simulink model "sdbe_10_11"  (R2012b)
settings: Solver=VariableStepDiscrete  SolverMode=SingleTasking  StartTime=0.0  StopTime=10000  RelTol=1e-3
PreLoadFcn:
  | counter_vals
undefined symbols (not defined in the file or in its folder): sfp
libraries: xbsIndex_r4 x8459, casper_library_misc x39, casper_library_delays x27, dspsigops x16, xps_library x10, r2dbe_vdif_lib x4, r2dbe_adc_lib x3, simulink x1
(part 61 of 72)

== system sdbe_10_11/get_data_from_pkt2/scope/quant11/is_positive ==
  d : Inport
  Reinterpret : xbsIndex_r4/Reinterpret  force_arith_type=on  arith_type=Unsigned  force_bin_pt=on  bin_pt=0  block_type=reinterpret
  not : xbsIndex_r4/Inverter  en=off  latency=0  dbl_ovrd=off  block_type=inv
  sgn : xbsIndex_r4/Slice  nbits=1  boolean_output=off  mode=Upper Bit Location + Width  bit1=0  base1=MSB of Input  bit0=0  base0=LSB of Input  dbl_ovrd=off  block_type=slice
  q : Outport
  wires:
  sgn/1 -> not/1
  Reinterpret/1 -> sgn/1
  d/1 -> Reinterpret/1
  not/1 -> q/1

== system sdbe_10_11/get_data_from_pkt2/scope/quant12/is_positive ==
  d : Inport
  Reinterpret : xbsIndex_r4/Reinterpret  force_arith_type=on  arith_type=Unsigned  force_bin_pt=on  bin_pt=0  block_type=reinterpret
  not : xbsIndex_r4/Inverter  en=off  latency=0  dbl_ovrd=off  block_type=inv
  sgn : xbsIndex_r4/Slice  nbits=1  boolean_output=off  mode=Upper Bit Location + Width  bit1=0  base1=MSB of Input  bit0=0  base0=LSB of Input  dbl_ovrd=off  block_type=slice
  q : Outport
  wires:
  not/1 -> q/1
  d/1 -> Reinterpret/1
  Reinterpret/1 -> sgn/1
  sgn/1 -> not/1

== system sdbe_10_11/get_data_from_pkt2/scope/quant13/is_positive ==
  d : Inport
  Reinterpret : xbsIndex_r4/Reinterpret  force_arith_type=on  arith_type=Unsigned  force_bin_pt=on  bin_pt=0  block_type=reinterpret
  not : xbsIndex_r4/Inverter  en=off  latency=0  dbl_ovrd=off  block_type=inv
  sgn : xbsIndex_r4/Slice  nbits=1  boolean_output=off  mode=Upper Bit Location + Width  bit1=0  base1=MSB of Input  bit0=0  base0=LSB of Input  dbl_ovrd=off  block_type=slice
  q : Outport
  wires:
  sgn/1 -> not/1
  Reinterpret/1 -> sgn/1
  d/1 -> Reinterpret/1
  not/1 -> q/1

== system sdbe_10_11/get_data_from_pkt2/scope/quant14/is_positive ==
  d : Inport
  Reinterpret : xbsIndex_r4/Reinterpret  force_arith_type=on  arith_type=Unsigned  force_bin_pt=on  bin_pt=0  block_type=reinterpret
  not : xbsIndex_r4/Inverter  en=off  latency=0  dbl_ovrd=off  block_type=inv
  sgn : xbsIndex_r4/Slice  nbits=1  boolean_output=off  mode=Upper Bit Location + Width  bit1=0  base1=MSB of Input  bit0=0  base0=LSB of Input  dbl_ovrd=off  block_type=slice
  q : Outport
  wires:
  sgn/1 -> not/1
  Reinterpret/1 -> sgn/1
  d/1 -> Reinterpret/1
  not/1 -> q/1

== system sdbe_10_11/get_data_from_pkt2/scope/quant15/is_positive ==
  d : Inport
  Reinterpret : xbsIndex_r4/Reinterpret  force_arith_type=on  arith_type=Unsigned  force_bin_pt=on  bin_pt=0  block_type=reinterpret
  not : xbsIndex_r4/Inverter  en=off  latency=0  dbl_ovrd=off  block_type=inv
  sgn : xbsIndex_r4/Slice  nbits=1  boolean_output=off  mode=Upper Bit Location + Width  bit1=0  base1=MSB of Input  bit0=0  base0=LSB of Input  dbl_ovrd=off  block_type=slice
  q : Outport
  wires:
  not/1 -> q/1
  d/1 -> Reinterpret/1
  Reinterpret/1 -> sgn/1
  sgn/1 -> not/1

== system sdbe_10_11/get_data_from_pkt2/scope/quant2/is_positive ==
  d : Inport
  Reinterpret : xbsIndex_r4/Reinterpret  force_arith_type=on  arith_type=Unsigned  force_bin_pt=on  bin_pt=0  block_type=reinterpret
  not : xbsIndex_r4/Inverter  en=off  latency=0  dbl_ovrd=off  block_type=inv
  sgn : xbsIndex_r4/Slice  nbits=1  boolean_output=off  mode=Upper Bit Location + Width  bit1=0  base1=MSB of Input  bit0=0  base0=LSB of Input  dbl_ovrd=off  block_type=slice
  q : Outport
  wires:
  sgn/1 -> not/1
  Reinterpret/1 -> sgn/1
  d/1 -> Reinterpret/1
  not/1 -> q/1

== system sdbe_10_11/get_data_from_pkt2/scope/quant3/is_positive ==
  d : Inport
  Reinterpret : xbsIndex_r4/Reinterpret  force_arith_type=on  arith_type=Unsigned  force_bin_pt=on  bin_pt=0  block_type=reinterpret
  not : xbsIndex_r4/Inverter  en=off  latency=0  dbl_ovrd=off  block_type=inv
  sgn : xbsIndex_r4/Slice  nbits=1  boolean_output=off  mode=Upper Bit Location + Width  bit1=0  base1=MSB of Input  bit0=0  base0=LSB of Input  dbl_ovrd=off  block_type=slice
  q : Outport
  wires:
  not/1 -> q/1
  d/1 -> Reinterpret/1
  Reinterpret/1 -> sgn/1
  sgn/1 -> not/1

== system sdbe_10_11/get_data_from_pkt2/scope/quant4/is_positive ==
  d : Inport
  Reinterpret : xbsIndex_r4/Reinterpret  force_arith_type=on  arith_type=Unsigned  force_bin_pt=on  bin_pt=0  block_type=reinterpret
  not : xbsIndex_r4/Inverter  en=off  latency=0  dbl_ovrd=off  block_type=inv
  sgn : xbsIndex_r4/Slice  nbits=1  boolean_output=off  mode=Upper Bit Location + Width  bit1=0  base1=MSB of Input  bit0=0  base0=LSB of Input  dbl_ovrd=off  block_type=slice
  q : Outport
  wires:
  sgn/1 -> not/1
  Reinterpret/1 -> sgn/1
  d/1 -> Reinterpret/1
  not/1 -> q/1

== system sdbe_10_11/get_data_from_pkt2/scope/quant5/is_positive ==
  d : Inport
  Reinterpret : xbsIndex_r4/Reinterpret  force_arith_type=on  arith_type=Unsigned  force_bin_pt=on  bin_pt=0  block_type=reinterpret
  not : xbsIndex_r4/Inverter  en=off  latency=0  dbl_ovrd=off  block_type=inv
  sgn : xbsIndex_r4/Slice  nbits=1  boolean_output=off  mode=Upper Bit Location + Width  bit1=0  base1=MSB of Input  bit0=0  base0=LSB of Input  dbl_ovrd=off  block_type=slice
  q : Outport
  wires:
  not/1 -> q/1
  d/1 -> Reinterpret/1
  Reinterpret/1 -> sgn/1
  sgn/1 -> not/1

== system sdbe_10_11/get_data_from_pkt2/scope/quant6/is_positive ==
  d : Inport
  Reinterpret : xbsIndex_r4/Reinterpret  force_arith_type=on  arith_type=Unsigned  force_bin_pt=on  bin_pt=0  block_type=reinterpret
  not : xbsIndex_r4/Inverter  en=off  latency=0  dbl_ovrd=off  block_type=inv
  sgn : xbsIndex_r4/Slice  nbits=1  boolean_output=off  mode=Upper Bit Location + Width  bit1=0  base1=MSB of Input  bit0=0  base0=LSB of Input  dbl_ovrd=off  block_type=slice
  q : Outport
  wires:
  not/1 -> q/1
  d/1 -> Reinterpret/1
  Reinterpret/1 -> sgn/1
  sgn/1 -> not/1

== system sdbe_10_11/get_data_from_pkt2/scope/quant7/is_positive ==
  d : Inport
  Reinterpret : xbsIndex_r4/Reinterpret  force_arith_type=on  arith_type=Unsigned  force_bin_pt=on  bin_pt=0  block_type=reinterpret
  not : xbsIndex_r4/Inverter  en=off  latency=0  dbl_ovrd=off  block_type=inv
  sgn : xbsIndex_r4/Slice  nbits=1  boolean_output=off  mode=Upper Bit Location + Width  bit1=0  base1=MSB of Input  bit0=0  base0=LSB of Input  dbl_ovrd=off  block_type=slice
  q : Outport
  wires:
  sgn/1 -> not/1
  Reinterpret/1 -> sgn/1
  d/1 -> Reinterpret/1
  not/1 -> q/1

== system sdbe_10_11/get_data_from_pkt2/scope/quant8/is_positive ==
  d : Inport
  Reinterpret : xbsIndex_r4/Reinterpret  force_arith_type=on  arith_type=Unsigned  force_bin_pt=on  bin_pt=0  block_type=reinterpret
  not : xbsIndex_r4/Inverter  en=off  latency=0  dbl_ovrd=off  block_type=inv
  sgn : xbsIndex_r4/Slice  nbits=1  boolean_output=off  mode=Upper Bit Location + Width  bit1=0  base1=MSB of Input  bit0=0  base0=LSB of Input  dbl_ovrd=off  block_type=slice
  q : Outport
  wires:
  sgn/1 -> not/1
  Reinterpret/1 -> sgn/1
  d/1 -> Reinterpret/1
  not/1 -> q/1

== system sdbe_10_11/get_data_from_pkt2/scope/quant9/is_positive ==
  d : Inport
  Reinterpret : xbsIndex_r4/Reinterpret  force_arith_type=on  arith_type=Unsigned  force_bin_pt=on  bin_pt=0  block_type=reinterpret
  not : xbsIndex_r4/Inverter  en=off  latency=0  dbl_ovrd=off  block_type=inv
  sgn : xbsIndex_r4/Slice  nbits=1  boolean_output=off  mode=Upper Bit Location + Width  bit1=0  base1=MSB of Input  bit0=0  base0=LSB of Input  dbl_ovrd=off  block_type=slice
  q : Outport
  wires:
  not/1 -> q/1
  d/1 -> Reinterpret/1
  Reinterpret/1 -> sgn/1
  sgn/1 -> not/1

== system sdbe_10_11/get_data_from_pkt3/scope/quant0/is_positive ==
  d : Inport
  Reinterpret : xbsIndex_r4/Reinterpret  force_arith_type=on  arith_type=Unsigned  force_bin_pt=on  bin_pt=0  block_type=reinterpret
  not : xbsIndex_r4/Inverter  en=off  latency=0  dbl_ovrd=off  block_type=inv
  sgn : xbsIndex_r4/Slice  nbits=1  boolean_output=off  mode=Upper Bit Location + Width  bit1=0  base1=MSB of Input  bit0=0  base0=LSB of Input  dbl_ovrd=off  block_type=slice
  q : Outport
  wires:
  sgn/1 -> not/1
  Reinterpret/1 -> sgn/1
  d/1 -> Reinterpret/1
  not/1 -> q/1

== system sdbe_10_11/get_data_from_pkt3/scope/quant1/is_positive ==
  d : Inport
  Reinterpret : xbsIndex_r4/Reinterpret  force_arith_type=on  arith_type=Unsigned  force_bin_pt=on  bin_pt=0  block_type=reinterpret
  not : xbsIndex_r4/Inverter  en=off  latency=0  dbl_ovrd=off  block_type=inv
  sgn : xbsIndex_r4/Slice  nbits=1  boolean_output=off  mode=Upper Bit Location + Width  bit1=0  base1=MSB of Input  bit0=0  base0=LSB of Input  dbl_ovrd=off  block_type=slice
  q : Outport
  wires:
  not/1 -> q/1
  d/1 -> Reinterpret/1
  Reinterpret/1 -> sgn/1
  sgn/1 -> not/1

== system sdbe_10_11/get_data_from_pkt3/scope/quant10/is_positive ==
  d : Inport
  Reinterpret : xbsIndex_r4/Reinterpret  force_arith_type=on  arith_type=Unsigned  force_bin_pt=on  bin_pt=0  block_type=reinterpret
  not : xbsIndex_r4/Inverter  en=off  latency=0  dbl_ovrd=off  block_type=inv
  sgn : xbsIndex_r4/Slice  nbits=1  boolean_output=off  mode=Upper Bit Location + Width  bit1=0  base1=MSB of Input  bit0=0  base0=LSB of Input  dbl_ovrd=off  block_type=slice
  q : Outport
  wires:
  sgn/1 -> not/1
  Reinterpret/1 -> sgn/1
  d/1 -> Reinterpret/1
  not/1 -> q/1

== system sdbe_10_11/get_data_from_pkt3/scope/quant11/is_positive ==
  d : Inport
  Reinterpret : xbsIndex_r4/Reinterpret  force_arith_type=on  arith_type=Unsigned  force_bin_pt=on  bin_pt=0  block_type=reinterpret
  not : xbsIndex_r4/Inverter  en=off  latency=0  dbl_ovrd=off  block_type=inv
  sgn : xbsIndex_r4/Slice  nbits=1  boolean_output=off  mode=Upper Bit Location + Width  bit1=0  base1=MSB of Input  bit0=0  base0=LSB of Input  dbl_ovrd=off  block_type=slice
  q : Outport
  wires:
  not/1 -> q/1
  d/1 -> Reinterpret/1
  Reinterpret/1 -> sgn/1
  sgn/1 -> not/1

== system sdbe_10_11/get_data_from_pkt3/scope/quant12/is_positive ==
  d : Inport
  Reinterpret : xbsIndex_r4/Reinterpret  force_arith_type=on  arith_type=Unsigned  force_bin_pt=on  bin_pt=0  block_type=reinterpret
  not : xbsIndex_r4/Inverter  en=off  latency=0  dbl_ovrd=off  block_type=inv
  sgn : xbsIndex_r4/Slice  nbits=1  boolean_output=off  mode=Upper Bit Location + Width  bit1=0  base1=MSB of Input  bit0=0  base0=LSB of Input  dbl_ovrd=off  block_type=slice
  q : Outport
  wires:
  sgn/1 -> not/1
  Reinterpret/1 -> sgn/1
  d/1 -> Reinterpret/1
  not/1 -> q/1

== system sdbe_10_11/get_data_from_pkt3/scope/quant13/is_positive ==
  d : Inport
  Reinterpret : xbsIndex_r4/Reinterpret  force_arith_type=on  arith_type=Unsigned  force_bin_pt=on  bin_pt=0  block_type=reinterpret
  not : xbsIndex_r4/Inverter  en=off  latency=0  dbl_ovrd=off  block_type=inv
  sgn : xbsIndex_r4/Slice  nbits=1  boolean_output=off  mode=Upper Bit Location + Width  bit1=0  base1=MSB of Input  bit0=0  base0=LSB of Input  dbl_ovrd=off  block_type=slice
  q : Outport
  wires:
  not/1 -> q/1
  d/1 -> Reinterpret/1
  Reinterpret/1 -> sgn/1
  sgn/1 -> not/1

== system sdbe_10_11/get_data_from_pkt3/scope/quant14/is_positive ==
  d : Inport
  Reinterpret : xbsIndex_r4/Reinterpret  force_arith_type=on  arith_type=Unsigned  force_bin_pt=on  bin_pt=0  block_type=reinterpret
  not : xbsIndex_r4/Inverter  en=off  latency=0  dbl_ovrd=off  block_type=inv
  sgn : xbsIndex_r4/Slice  nbits=1  boolean_output=off  mode=Upper Bit Location + Width  bit1=0  base1=MSB of Input  bit0=0  base0=LSB of Input  dbl_ovrd=off  block_type=slice
  q : Outport
  wires:
  not/1 -> q/1
  d/1 -> Reinterpret/1
  Reinterpret/1 -> sgn/1
  sgn/1 -> not/1

== system sdbe_10_11/get_data_from_pkt3/scope/quant15/is_positive ==
  d : Inport
  Reinterpret : xbsIndex_r4/Reinterpret  force_arith_type=on  arith_type=Unsigned  force_bin_pt=on  bin_pt=0  block_type=reinterpret
  not : xbsIndex_r4/Inverter  en=off  latency=0  dbl_ovrd=off  block_type=inv
  sgn : xbsIndex_r4/Slice  nbits=1  boolean_output=off  mode=Upper Bit Location + Width  bit1=0  base1=MSB of Input  bit0=0  base0=LSB of Input  dbl_ovrd=off  block_type=slice
  q : Outport
  wires:
  sgn/1 -> not/1
  Reinterpret/1 -> sgn/1
  d/1 -> Reinterpret/1
  not/1 -> q/1

== system sdbe_10_11/get_data_from_pkt3/scope/quant2/is_positive ==
  d : Inport
  Reinterpret : xbsIndex_r4/Reinterpret  force_arith_type=on  arith_type=Unsigned  force_bin_pt=on  bin_pt=0  block_type=reinterpret
  not : xbsIndex_r4/Inverter  en=off  latency=0  dbl_ovrd=off  block_type=inv
  sgn : xbsIndex_r4/Slice  nbits=1  boolean_output=off  mode=Upper Bit Location + Width  bit1=0  base1=MSB of Input  bit0=0  base0=LSB of Input  dbl_ovrd=off  block_type=slice
  q : Outport
  wires:
  not/1 -> q/1
  d/1 -> Reinterpret/1
  Reinterpret/1 -> sgn/1
  sgn/1 -> not/1

== system sdbe_10_11/get_data_from_pkt3/scope/quant3/is_positive ==
  d : Inport
  Reinterpret : xbsIndex_r4/Reinterpret  force_arith_type=on  arith_type=Unsigned  force_bin_pt=on  bin_pt=0  block_type=reinterpret
  not : xbsIndex_r4/Inverter  en=off  latency=0  dbl_ovrd=off  block_type=inv
  sgn : xbsIndex_r4/Slice  nbits=1  boolean_output=off  mode=Upper Bit Location + Width  bit1=0  base1=MSB of Input  bit0=0  base0=LSB of Input  dbl_ovrd=off  block_type=slice
  q : Outport
  wires:
  sgn/1 -> not/1
  Reinterpret/1 -> sgn/1
  d/1 -> Reinterpret/1
  not/1 -> q/1

== system sdbe_10_11/get_data_from_pkt3/scope/quant4/is_positive ==
  d : Inport
  Reinterpret : xbsIndex_r4/Reinterpret  force_arith_type=on  arith_type=Unsigned  force_bin_pt=on  bin_pt=0  block_type=reinterpret
  not : xbsIndex_r4/Inverter  en=off  latency=0  dbl_ovrd=off  block_type=inv
  sgn : xbsIndex_r4/Slice  nbits=1  boolean_output=off  mode=Upper Bit Location + Width  bit1=0  base1=MSB of Input  bit0=0  base0=LSB of Input  dbl_ovrd=off  block_type=slice
  q : Outport
  wires:
  not/1 -> q/1
  d/1 -> Reinterpret/1
  Reinterpret/1 -> sgn/1
  sgn/1 -> not/1

== system sdbe_10_11/get_data_from_pkt3/scope/quant5/is_positive ==
  d : Inport
  Reinterpret : xbsIndex_r4/Reinterpret  force_arith_type=on  arith_type=Unsigned  force_bin_pt=on  bin_pt=0  block_type=reinterpret
  not : xbsIndex_r4/Inverter  en=off  latency=0  dbl_ovrd=off  block_type=inv
  sgn : xbsIndex_r4/Slice  nbits=1  boolean_output=off  mode=Upper Bit Location + Width  bit1=0  base1=MSB of Input  bit0=0  base0=LSB of Input  dbl_ovrd=off  block_type=slice
  q : Outport
  wires:
  sgn/1 -> not/1
  Reinterpret/1 -> sgn/1
  d/1 -> Reinterpret/1
  not/1 -> q/1

== system sdbe_10_11/get_data_from_pkt3/scope/quant6/is_positive ==
  d : Inport
  Reinterpret : xbsIndex_r4/Reinterpret  force_arith_type=on  arith_type=Unsigned  force_bin_pt=on  bin_pt=0  block_type=reinterpret
  not : xbsIndex_r4/Inverter  en=off  latency=0  dbl_ovrd=off  block_type=inv
  sgn : xbsIndex_r4/Slice  nbits=1  boolean_output=off  mode=Upper Bit Location + Width  bit1=0  base1=MSB of Input  bit0=0  base0=LSB of Input  dbl_ovrd=off  block_type=slice
  q : Outport
  wires:
  sgn/1 -> not/1
  Reinterpret/1 -> sgn/1
  d/1 -> Reinterpret/1
  not/1 -> q/1

== system sdbe_10_11/get_data_from_pkt3/scope/quant7/is_positive ==
  d : Inport
  Reinterpret : xbsIndex_r4/Reinterpret  force_arith_type=on  arith_type=Unsigned  force_bin_pt=on  bin_pt=0  block_type=reinterpret
  not : xbsIndex_r4/Inverter  en=off  latency=0  dbl_ovrd=off  block_type=inv
  sgn : xbsIndex_r4/Slice  nbits=1  boolean_output=off  mode=Upper Bit Location + Width  bit1=0  base1=MSB of Input  bit0=0  base0=LSB of Input  dbl_ovrd=off  block_type=slice
  q : Outport
  wires:
  not/1 -> q/1
  d/1 -> Reinterpret/1
  Reinterpret/1 -> sgn/1
  sgn/1 -> not/1

== system sdbe_10_11/get_data_from_pkt3/scope/quant8/is_positive ==
  d : Inport
  Reinterpret : xbsIndex_r4/Reinterpret  force_arith_type=on  arith_type=Unsigned  force_bin_pt=on  bin_pt=0  block_type=reinterpret
  not : xbsIndex_r4/Inverter  en=off  latency=0  dbl_ovrd=off  block_type=inv
  sgn : xbsIndex_r4/Slice  nbits=1  boolean_output=off  mode=Upper Bit Location + Width  bit1=0  base1=MSB of Input  bit0=0  base0=LSB of Input  dbl_ovrd=off  block_type=slice
  q : Outport
  wires:
  not/1 -> q/1
  d/1 -> Reinterpret/1
  Reinterpret/1 -> sgn/1
  sgn/1 -> not/1

== system sdbe_10_11/get_data_from_pkt3/scope/quant9/is_positive ==
  d : Inport
  Reinterpret : xbsIndex_r4/Reinterpret  force_arith_type=on  arith_type=Unsigned  force_bin_pt=on  bin_pt=0  block_type=reinterpret
  not : xbsIndex_r4/Inverter  en=off  latency=0  dbl_ovrd=off  block_type=inv
  sgn : xbsIndex_r4/Slice  nbits=1  boolean_output=off  mode=Upper Bit Location + Width  bit1=0  base1=MSB of Input  bit0=0  base0=LSB of Input  dbl_ovrd=off  block_type=slice
  q : Outport
  wires:
  sgn/1 -> not/1
  Reinterpret/1 -> sgn/1
  d/1 -> Reinterpret/1
  not/1 -> q/1

== system sdbe_10_11/quantize_0/vlbi_2bit/quant/invcat ==
  b : Inport
  Concat : xbsIndex_r4/Concat  num_inputs=2  dbl_ovrd=off  block_type=concat
  Inverter : xbsIndex_r4/Inverter  en=off  latency=0  dbl_ovrd=off  block_type=inv
  bb : Outport
  wires:
  b/1 -> Inverter/1, Concat/2
  Inverter/1 -> Concat/1
  Concat/1 -> bb/1

== system sdbe_10_11/quantize_0/vlbi_2bit/quant/is_positive ==
  d : Inport
  Reinterpret : xbsIndex_r4/Reinterpret  force_arith_type=on  arith_type=Unsigned  force_bin_pt=on  bin_pt=0  block_type=reinterpret
  not : xbsIndex_r4/Inverter  en=off  latency=0  dbl_ovrd=off  block_type=inv
  sgn : xbsIndex_r4/Slice  nbits=1  boolean_output=off  mode=Upper Bit Location + Width  bit1=0  base1=MSB of Input  bit0=0  base0=LSB of Input  dbl_ovrd=off  block_type=slice
  q : Outport
  wires:
  not/1 -> q/1
  d/1 -> Reinterpret/1
  Reinterpret/1 -> sgn/1
  sgn/1 -> not/1

== system sdbe_10_11/quantize_0/vlbi_2bit/quant1/invcat ==
  b : Inport
  Concat : xbsIndex_r4/Concat  num_inputs=2  dbl_ovrd=off  block_type=concat
  Inverter : xbsIndex_r4/Inverter  en=off  latency=0  dbl_ovrd=off  block_type=inv
  bb : Outport
  wires:
  Concat/1 -> bb/1
  Inverter/1 -> Concat/1
  b/1 -> Concat/2, Inverter/1

== system sdbe_10_11/quantize_0/vlbi_2bit/quant1/is_positive ==
  d : Inport
  Reinterpret : xbsIndex_r4/Reinterpret  force_arith_type=on  arith_type=Unsigned  force_bin_pt=on  bin_pt=0  block_type=reinterpret
  not : xbsIndex_r4/Inverter  en=off  latency=0  dbl_ovrd=off  block_type=inv
  sgn : xbsIndex_r4/Slice  nbits=1  boolean_output=off  mode=Upper Bit Location + Width  bit1=0  base1=MSB of Input  bit0=0  base0=LSB of Input  dbl_ovrd=off  block_type=slice
  q : Outport
  wires:
  sgn/1 -> not/1
  Reinterpret/1 -> sgn/1
  d/1 -> Reinterpret/1
  not/1 -> q/1

== system sdbe_10_11/quantize_0/vlbi_2bit/quant10/invcat ==
  b : Inport
  Concat : xbsIndex_r4/Concat  num_inputs=2  dbl_ovrd=off  block_type=concat
  Inverter : xbsIndex_r4/Inverter  en=off  latency=0  dbl_ovrd=off  block_type=inv
  bb : Outport
  wires:
  b/1 -> Inverter/1, Concat/2
  Inverter/1 -> Concat/1
  Concat/1 -> bb/1

== system sdbe_10_11/quantize_0/vlbi_2bit/quant10/is_positive ==
  d : Inport
  Reinterpret : xbsIndex_r4/Reinterpret  force_arith_type=on  arith_type=Unsigned  force_bin_pt=on  bin_pt=0  block_type=reinterpret
  not : xbsIndex_r4/Inverter  en=off  latency=0  dbl_ovrd=off  block_type=inv
  sgn : xbsIndex_r4/Slice  nbits=1  boolean_output=off  mode=Upper Bit Location + Width  bit1=0  base1=MSB of Input  bit0=0  base0=LSB of Input  dbl_ovrd=off  block_type=slice
  q : Outport
  wires:
  not/1 -> q/1
  d/1 -> Reinterpret/1
  Reinterpret/1 -> sgn/1
  sgn/1 -> not/1

== system sdbe_10_11/quantize_0/vlbi_2bit/quant11/invcat ==
  b : Inport
  Concat : xbsIndex_r4/Concat  num_inputs=2  dbl_ovrd=off  block_type=concat
  Inverter : xbsIndex_r4/Inverter  en=off  latency=0  dbl_ovrd=off  block_type=inv
  bb : Outport
  wires:
  Concat/1 -> bb/1
  Inverter/1 -> Concat/1
  b/1 -> Concat/2, Inverter/1

== system sdbe_10_11/quantize_0/vlbi_2bit/quant11/is_positive ==
  d : Inport
  Reinterpret : xbsIndex_r4/Reinterpret  force_arith_type=on  arith_type=Unsigned  force_bin_pt=on  bin_pt=0  block_type=reinterpret
  not : xbsIndex_r4/Inverter  en=off  latency=0  dbl_ovrd=off  block_type=inv
  sgn : xbsIndex_r4/Slice  nbits=1  boolean_output=off  mode=Upper Bit Location + Width  bit1=0  base1=MSB of Input  bit0=0  base0=LSB of Input  dbl_ovrd=off  block_type=slice
  q : Outport
  wires:
  sgn/1 -> not/1
  Reinterpret/1 -> sgn/1
  d/1 -> Reinterpret/1
  not/1 -> q/1

== system sdbe_10_11/quantize_0/vlbi_2bit/quant12/invcat ==
  b : Inport
  Concat : xbsIndex_r4/Concat  num_inputs=2  dbl_ovrd=off  block_type=concat
  Inverter : xbsIndex_r4/Inverter  en=off  latency=0  dbl_ovrd=off  block_type=inv
  bb : Outport
  wires:
  b/1 -> Inverter/1, Concat/2
  Inverter/1 -> Concat/1
  Concat/1 -> bb/1

== system sdbe_10_11/quantize_0/vlbi_2bit/quant12/is_positive ==
  d : Inport
  Reinterpret : xbsIndex_r4/Reinterpret  force_arith_type=on  arith_type=Unsigned  force_bin_pt=on  bin_pt=0  block_type=reinterpret
  not : xbsIndex_r4/Inverter  en=off  latency=0  dbl_ovrd=off  block_type=inv
  sgn : xbsIndex_r4/Slice  nbits=1  boolean_output=off  mode=Upper Bit Location + Width  bit1=0  base1=MSB of Input  bit0=0  base0=LSB of Input  dbl_ovrd=off  block_type=slice
  q : Outport
  wires:
  not/1 -> q/1
  d/1 -> Reinterpret/1
  Reinterpret/1 -> sgn/1
  sgn/1 -> not/1

== system sdbe_10_11/quantize_0/vlbi_2bit/quant13/invcat ==
  b : Inport
  Concat : xbsIndex_r4/Concat  num_inputs=2  dbl_ovrd=off  block_type=concat
  Inverter : xbsIndex_r4/Inverter  en=off  latency=0  dbl_ovrd=off  block_type=inv
  bb : Outport
  wires:
  Concat/1 -> bb/1
  Inverter/1 -> Concat/1
  b/1 -> Concat/2, Inverter/1

== system sdbe_10_11/quantize_0/vlbi_2bit/quant13/is_positive ==
  d : Inport
  Reinterpret : xbsIndex_r4/Reinterpret  force_arith_type=on  arith_type=Unsigned  force_bin_pt=on  bin_pt=0  block_type=reinterpret
  not : xbsIndex_r4/Inverter  en=off  latency=0  dbl_ovrd=off  block_type=inv
  sgn : xbsIndex_r4/Slice  nbits=1  boolean_output=off  mode=Upper Bit Location + Width  bit1=0  base1=MSB of Input  bit0=0  base0=LSB of Input  dbl_ovrd=off  block_type=slice
  q : Outport
  wires:
  sgn/1 -> not/1
  Reinterpret/1 -> sgn/1
  d/1 -> Reinterpret/1
  not/1 -> q/1

== system sdbe_10_11/quantize_0/vlbi_2bit/quant14/invcat ==
  b : Inport
  Concat : xbsIndex_r4/Concat  num_inputs=2  dbl_ovrd=off  block_type=concat
  Inverter : xbsIndex_r4/Inverter  en=off  latency=0  dbl_ovrd=off  block_type=inv
  bb : Outport
  wires:
  b/1 -> Inverter/1, Concat/2
  Inverter/1 -> Concat/1
  Concat/1 -> bb/1

== system sdbe_10_11/quantize_0/vlbi_2bit/quant14/is_positive ==
  d : Inport
  Reinterpret : xbsIndex_r4/Reinterpret  force_arith_type=on  arith_type=Unsigned  force_bin_pt=on  bin_pt=0  block_type=reinterpret
  not : xbsIndex_r4/Inverter  en=off  latency=0  dbl_ovrd=off  block_type=inv
  sgn : xbsIndex_r4/Slice  nbits=1  boolean_output=off  mode=Upper Bit Location + Width  bit1=0  base1=MSB of Input  bit0=0  base0=LSB of Input  dbl_ovrd=off  block_type=slice
  q : Outport
  wires:
  not/1 -> q/1
  d/1 -> Reinterpret/1
  Reinterpret/1 -> sgn/1
  sgn/1 -> not/1

== system sdbe_10_11/quantize_0/vlbi_2bit/quant15/invcat ==
  b : Inport
  Concat : xbsIndex_r4/Concat  num_inputs=2  dbl_ovrd=off  block_type=concat
  Inverter : xbsIndex_r4/Inverter  en=off  latency=0  dbl_ovrd=off  block_type=inv
  bb : Outport
  wires:
  Concat/1 -> bb/1
  Inverter/1 -> Concat/1
  b/1 -> Concat/2, Inverter/1

== system sdbe_10_11/quantize_0/vlbi_2bit/quant15/is_positive ==
  d : Inport
  Reinterpret : xbsIndex_r4/Reinterpret  force_arith_type=on  arith_type=Unsigned  force_bin_pt=on  bin_pt=0  block_type=reinterpret
  not : xbsIndex_r4/Inverter  en=off  latency=0  dbl_ovrd=off  block_type=inv
  sgn : xbsIndex_r4/Slice  nbits=1  boolean_output=off  mode=Upper Bit Location + Width  bit1=0  base1=MSB of Input  bit0=0  base0=LSB of Input  dbl_ovrd=off  block_type=slice
  q : Outport
  wires:
  sgn/1 -> not/1
  Reinterpret/1 -> sgn/1
  d/1 -> Reinterpret/1
  not/1 -> q/1

== system sdbe_10_11/quantize_0/vlbi_2bit/quant2/invcat ==
  b : Inport
  Concat : xbsIndex_r4/Concat  num_inputs=2  dbl_ovrd=off  block_type=concat
  Inverter : xbsIndex_r4/Inverter  en=off  latency=0  dbl_ovrd=off  block_type=inv
  bb : Outport
  wires:
  b/1 -> Inverter/1, Concat/2
  Inverter/1 -> Concat/1
  Concat/1 -> bb/1

== system sdbe_10_11/quantize_0/vlbi_2bit/quant2/is_positive ==
  d : Inport
  Reinterpret : xbsIndex_r4/Reinterpret  force_arith_type=on  arith_type=Unsigned  force_bin_pt=on  bin_pt=0  block_type=reinterpret
  not : xbsIndex_r4/Inverter  en=off  latency=0  dbl_ovrd=off  block_type=inv
  sgn : xbsIndex_r4/Slice  nbits=1  boolean_output=off  mode=Upper Bit Location + Width  bit1=0  base1=MSB of Input  bit0=0  base0=LSB of Input  dbl_ovrd=off  block_type=slice
  q : Outport
  wires:
  not/1 -> q/1
  d/1 -> Reinterpret/1
  Reinterpret/1 -> sgn/1
  sgn/1 -> not/1

== system sdbe_10_11/quantize_0/vlbi_2bit/quant3/invcat ==
  b : Inport
  Concat : xbsIndex_r4/Concat  num_inputs=2  dbl_ovrd=off  block_type=concat
  Inverter : xbsIndex_r4/Inverter  en=off  latency=0  dbl_ovrd=off  block_type=inv
  bb : Outport
  wires:
  Concat/1 -> bb/1
  Inverter/1 -> Concat/1
  b/1 -> Concat/2, Inverter/1

== system sdbe_10_11/quantize_0/vlbi_2bit/quant3/is_positive ==
  d : Inport
  Reinterpret : xbsIndex_r4/Reinterpret  force_arith_type=on  arith_type=Unsigned  force_bin_pt=on  bin_pt=0  block_type=reinterpret
  not : xbsIndex_r4/Inverter  en=off  latency=0  dbl_ovrd=off  block_type=inv
  sgn : xbsIndex_r4/Slice  nbits=1  boolean_output=off  mode=Upper Bit Location + Width  bit1=0  base1=MSB of Input  bit0=0  base0=LSB of Input  dbl_ovrd=off  block_type=slice
  q : Outport
  wires:
  sgn/1 -> not/1
  Reinterpret/1 -> sgn/1
  d/1 -> Reinterpret/1
  not/1 -> q/1

== system sdbe_10_11/quantize_0/vlbi_2bit/quant4/invcat ==
  b : Inport
  Concat : xbsIndex_r4/Concat  num_inputs=2  dbl_ovrd=off  block_type=concat
  Inverter : xbsIndex_r4/Inverter  en=off  latency=0  dbl_ovrd=off  block_type=inv
  bb : Outport
  wires:
  b/1 -> Inverter/1, Concat/2
  Inverter/1 -> Concat/1
  Concat/1 -> bb/1

== system sdbe_10_11/quantize_0/vlbi_2bit/quant4/is_positive ==
  d : Inport
  Reinterpret : xbsIndex_r4/Reinterpret  force_arith_type=on  arith_type=Unsigned  force_bin_pt=on  bin_pt=0  block_type=reinterpret
  not : xbsIndex_r4/Inverter  en=off  latency=0  dbl_ovrd=off  block_type=inv
  sgn : xbsIndex_r4/Slice  nbits=1  boolean_output=off  mode=Upper Bit Location + Width  bit1=0  base1=MSB of Input  bit0=0  base0=LSB of Input  dbl_ovrd=off  block_type=slice
  q : Outport
  wires:
  not/1 -> q/1
  d/1 -> Reinterpret/1
  Reinterpret/1 -> sgn/1
  sgn/1 -> not/1

== system sdbe_10_11/quantize_0/vlbi_2bit/quant5/invcat ==
  b : Inport
  Concat : xbsIndex_r4/Concat  num_inputs=2  dbl_ovrd=off  block_type=concat
  Inverter : xbsIndex_r4/Inverter  en=off  latency=0  dbl_ovrd=off  block_type=inv
  bb : Outport
  wires:
  Concat/1 -> bb/1
  Inverter/1 -> Concat/1
  b/1 -> Concat/2, Inverter/1

== system sdbe_10_11/quantize_0/vlbi_2bit/quant5/is_positive ==
  d : Inport
  Reinterpret : xbsIndex_r4/Reinterpret  force_arith_type=on  arith_type=Unsigned  force_bin_pt=on  bin_pt=0  block_type=reinterpret
  not : xbsIndex_r4/Inverter  en=off  latency=0  dbl_ovrd=off  block_type=inv
  sgn : xbsIndex_r4/Slice  nbits=1  boolean_output=off  mode=Upper Bit Location + Width  bit1=0  base1=MSB of Input  bit0=0  base0=LSB of Input  dbl_ovrd=off  block_type=slice
  q : Outport
  wires:
  sgn/1 -> not/1
  Reinterpret/1 -> sgn/1
  d/1 -> Reinterpret/1
  not/1 -> q/1

== system sdbe_10_11/quantize_0/vlbi_2bit/quant6/invcat ==
  b : Inport
  Concat : xbsIndex_r4/Concat  num_inputs=2  dbl_ovrd=off  block_type=concat
  Inverter : xbsIndex_r4/Inverter  en=off  latency=0  dbl_ovrd=off  block_type=inv
  bb : Outport
  wires:
  b/1 -> Inverter/1, Concat/2
  Inverter/1 -> Concat/1
  Concat/1 -> bb/1

== system sdbe_10_11/quantize_0/vlbi_2bit/quant6/is_positive ==
  d : Inport
  Reinterpret : xbsIndex_r4/Reinterpret  force_arith_type=on  arith_type=Unsigned  force_bin_pt=on  bin_pt=0  block_type=reinterpret
  not : xbsIndex_r4/Inverter  en=off  latency=0  dbl_ovrd=off  block_type=inv
  sgn : xbsIndex_r4/Slice  nbits=1  boolean_output=off  mode=Upper Bit Location + Width  bit1=0  base1=MSB of Input  bit0=0  base0=LSB of Input  dbl_ovrd=off  block_type=slice
  q : Outport
  wires:
  not/1 -> q/1
  d/1 -> Reinterpret/1
  Reinterpret/1 -> sgn/1
  sgn/1 -> not/1

== system sdbe_10_11/quantize_0/vlbi_2bit/quant7/invcat ==
  b : Inport
  Concat : xbsIndex_r4/Concat  num_inputs=2  dbl_ovrd=off  block_type=concat
  Inverter : xbsIndex_r4/Inverter  en=off  latency=0  dbl_ovrd=off  block_type=inv
  bb : Outport
  wires:
  Concat/1 -> bb/1
  Inverter/1 -> Concat/1
  b/1 -> Concat/2, Inverter/1

== system sdbe_10_11/quantize_0/vlbi_2bit/quant7/is_positive ==
  d : Inport
  Reinterpret : xbsIndex_r4/Reinterpret  force_arith_type=on  arith_type=Unsigned  force_bin_pt=on  bin_pt=0  block_type=reinterpret
  not : xbsIndex_r4/Inverter  en=off  latency=0  dbl_ovrd=off  block_type=inv
  sgn : xbsIndex_r4/Slice  nbits=1  boolean_output=off  mode=Upper Bit Location + Width  bit1=0  base1=MSB of Input  bit0=0  base0=LSB of Input  dbl_ovrd=off  block_type=slice
  q : Outport
  wires:
  sgn/1 -> not/1
  Reinterpret/1 -> sgn/1
  d/1 -> Reinterpret/1
  not/1 -> q/1

== system sdbe_10_11/quantize_0/vlbi_2bit/quant8/invcat ==
  b : Inport
  Concat : xbsIndex_r4/Concat  num_inputs=2  dbl_ovrd=off  block_type=concat
  Inverter : xbsIndex_r4/Inverter  en=off  latency=0  dbl_ovrd=off  block_type=inv
  bb : Outport
  wires:
  b/1 -> Inverter/1, Concat/2
  Inverter/1 -> Concat/1
  Concat/1 -> bb/1

== system sdbe_10_11/quantize_0/vlbi_2bit/quant8/is_positive ==
  d : Inport
  Reinterpret : xbsIndex_r4/Reinterpret  force_arith_type=on  arith_type=Unsigned  force_bin_pt=on  bin_pt=0  block_type=reinterpret
  not : xbsIndex_r4/Inverter  en=off  latency=0  dbl_ovrd=off  block_type=inv
  sgn : xbsIndex_r4/Slice  nbits=1  boolean_output=off  mode=Upper Bit Location + Width  bit1=0  base1=MSB of Input  bit0=0  base0=LSB of Input  dbl_ovrd=off  block_type=slice
  q : Outport
  wires:
  not/1 -> q/1
  d/1 -> Reinterpret/1
  Reinterpret/1 -> sgn/1
  sgn/1 -> not/1

== system sdbe_10_11/quantize_0/vlbi_2bit/quant9/invcat ==
  b : Inport
  Concat : xbsIndex_r4/Concat  num_inputs=2  dbl_ovrd=off  block_type=concat
  Inverter : xbsIndex_r4/Inverter  en=off  latency=0  dbl_ovrd=off  block_type=inv
  bb : Outport
  wires:
  Concat/1 -> bb/1
  Inverter/1 -> Concat/1
  b/1 -> Concat/2, Inverter/1

== system sdbe_10_11/quantize_0/vlbi_2bit/quant9/is_positive ==
  d : Inport
  Reinterpret : xbsIndex_r4/Reinterpret  force_arith_type=on  arith_type=Unsigned  force_bin_pt=on  bin_pt=0  block_type=reinterpret
  not : xbsIndex_r4/Inverter  en=off  latency=0  dbl_ovrd=off  block_type=inv
  sgn : xbsIndex_r4/Slice  nbits=1  boolean_output=off  mode=Upper Bit Location + Width  bit1=0  base1=MSB of Input  bit0=0  base0=LSB of Input  dbl_ovrd=off  block_type=slice
  q : Outport
  wires:
  sgn/1 -> not/1
  Reinterpret/1 -> sgn/1
  d/1 -> Reinterpret/1
  not/1 -> q/1

== system sdbe_10_11/quantize_1/vlbi_2bit/quant/invcat ==
  b : Inport
  Concat : xbsIndex_r4/Concat  num_inputs=2  dbl_ovrd=off  block_type=concat
  Inverter : xbsIndex_r4/Inverter  en=off  latency=0  dbl_ovrd=off  block_type=inv
  bb : Outport
  wires:
  Concat/1 -> bb/1
  Inverter/1 -> Concat/1
  b/1 -> Concat/2, Inverter/1

== system sdbe_10_11/quantize_1/vlbi_2bit/quant/is_positive ==
  d : Inport
  Reinterpret : xbsIndex_r4/Reinterpret  force_arith_type=on  arith_type=Unsigned  force_bin_pt=on  bin_pt=0  block_type=reinterpret
  not : xbsIndex_r4/Inverter  en=off  latency=0  dbl_ovrd=off  block_type=inv
  sgn : xbsIndex_r4/Slice  nbits=1  boolean_output=off  mode=Upper Bit Location + Width  bit1=0  base1=MSB of Input  bit0=0  base0=LSB of Input  dbl_ovrd=off  block_type=slice
  q : Outport
  wires:
  sgn/1 -> not/1
  Reinterpret/1 -> sgn/1
  d/1 -> Reinterpret/1
  not/1 -> q/1

== system sdbe_10_11/quantize_1/vlbi_2bit/quant1/invcat ==
  b : Inport
  Concat : xbsIndex_r4/Concat  num_inputs=2  dbl_ovrd=off  block_type=concat
  Inverter : xbsIndex_r4/Inverter  en=off  latency=0  dbl_ovrd=off  block_type=inv
  bb : Outport
  wires:
  b/1 -> Inverter/1, Concat/2
  Inverter/1 -> Concat/1
  Concat/1 -> bb/1

== system sdbe_10_11/quantize_1/vlbi_2bit/quant1/is_positive ==
  d : Inport
  Reinterpret : xbsIndex_r4/Reinterpret  force_arith_type=on  arith_type=Unsigned  force_bin_pt=on  bin_pt=0  block_type=reinterpret
  not : xbsIndex_r4/Inverter  en=off  latency=0  dbl_ovrd=off  block_type=inv
  sgn : xbsIndex_r4/Slice  nbits=1  boolean_output=off  mode=Upper Bit Location + Width  bit1=0  base1=MSB of Input  bit0=0  base0=LSB of Input  dbl_ovrd=off  block_type=slice
  q : Outport
  wires:
  not/1 -> q/1
  d/1 -> Reinterpret/1
  Reinterpret/1 -> sgn/1
  sgn/1 -> not/1

== system sdbe_10_11/quantize_1/vlbi_2bit/quant10/invcat ==
  b : Inport
  Concat : xbsIndex_r4/Concat  num_inputs=2  dbl_ovrd=off  block_type=concat
  Inverter : xbsIndex_r4/Inverter  en=off  latency=0  dbl_ovrd=off  block_type=inv
  bb : Outport
  wires:
  Concat/1 -> bb/1
  Inverter/1 -> Concat/1
  b/1 -> Concat/2, Inverter/1

== system sdbe_10_11/quantize_1/vlbi_2bit/quant10/is_positive ==
  d : Inport
  Reinterpret : xbsIndex_r4/Reinterpret  force_arith_type=on  arith_type=Unsigned  force_bin_pt=on  bin_pt=0  block_type=reinterpret
  not : xbsIndex_r4/Inverter  en=off  latency=0  dbl_ovrd=off  block_type=inv
  sgn : xbsIndex_r4/Slice  nbits=1  boolean_output=off  mode=Upper Bit Location + Width  bit1=0  base1=MSB of Input  bit0=0  base0=LSB of Input  dbl_ovrd=off  block_type=slice
  q : Outport
  wires:
  sgn/1 -> not/1
  Reinterpret/1 -> sgn/1
  d/1 -> Reinterpret/1
  not/1 -> q/1

== system sdbe_10_11/quantize_1/vlbi_2bit/quant11/invcat ==
  b : Inport
  Concat : xbsIndex_r4/Concat  num_inputs=2  dbl_ovrd=off  block_type=concat
  Inverter : xbsIndex_r4/Inverter  en=off  latency=0  dbl_ovrd=off  block_type=inv
  bb : Outport
  wires:
  b/1 -> Inverter/1, Concat/2
  Inverter/1 -> Concat/1
  Concat/1 -> bb/1

== system sdbe_10_11/quantize_1/vlbi_2bit/quant11/is_positive ==
  d : Inport
  Reinterpret : xbsIndex_r4/Reinterpret  force_arith_type=on  arith_type=Unsigned  force_bin_pt=on  bin_pt=0  block_type=reinterpret
  not : xbsIndex_r4/Inverter  en=off  latency=0  dbl_ovrd=off  block_type=inv
  sgn : xbsIndex_r4/Slice  nbits=1  boolean_output=off  mode=Upper Bit Location + Width  bit1=0  base1=MSB of Input  bit0=0  base0=LSB of Input  dbl_ovrd=off  block_type=slice
  q : Outport
  wires:
  not/1 -> q/1
  d/1 -> Reinterpret/1
  Reinterpret/1 -> sgn/1
  sgn/1 -> not/1

== system sdbe_10_11/quantize_1/vlbi_2bit/quant12/invcat ==
  b : Inport
  Concat : xbsIndex_r4/Concat  num_inputs=2  dbl_ovrd=off  block_type=concat
  Inverter : xbsIndex_r4/Inverter  en=off  latency=0  dbl_ovrd=off  block_type=inv
  bb : Outport
  wires:
  Concat/1 -> bb/1
  Inverter/1 -> Concat/1
  b/1 -> Concat/2, Inverter/1

== system sdbe_10_11/quantize_1/vlbi_2bit/quant12/is_positive ==
  d : Inport
  Reinterpret : xbsIndex_r4/Reinterpret  force_arith_type=on  arith_type=Unsigned  force_bin_pt=on  bin_pt=0  block_type=reinterpret
  not : xbsIndex_r4/Inverter  en=off  latency=0  dbl_ovrd=off  block_type=inv
  sgn : xbsIndex_r4/Slice  nbits=1  boolean_output=off  mode=Upper Bit Location + Width  bit1=0  base1=MSB of Input  bit0=0  base0=LSB of Input  dbl_ovrd=off  block_type=slice
  q : Outport
  wires:
  sgn/1 -> not/1
  Reinterpret/1 -> sgn/1
  d/1 -> Reinterpret/1
  not/1 -> q/1

== system sdbe_10_11/quantize_1/vlbi_2bit/quant13/invcat ==
  b : Inport
  Concat : xbsIndex_r4/Concat  num_inputs=2  dbl_ovrd=off  block_type=concat
  Inverter : xbsIndex_r4/Inverter  en=off  latency=0  dbl_ovrd=off  block_type=inv
  bb : Outport
  wires:
  b/1 -> Inverter/1, Concat/2
  Inverter/1 -> Concat/1
  Concat/1 -> bb/1

== system sdbe_10_11/quantize_1/vlbi_2bit/quant13/is_positive ==
  d : Inport
  Reinterpret : xbsIndex_r4/Reinterpret  force_arith_type=on  arith_type=Unsigned  force_bin_pt=on  bin_pt=0  block_type=reinterpret
  not : xbsIndex_r4/Inverter  en=off  latency=0  dbl_ovrd=off  block_type=inv
  sgn : xbsIndex_r4/Slice  nbits=1  boolean_output=off  mode=Upper Bit Location + Width  bit1=0  base1=MSB of Input  bit0=0  base0=LSB of Input  dbl_ovrd=off  block_type=slice
  q : Outport
  wires:
  not/1 -> q/1
  d/1 -> Reinterpret/1
  Reinterpret/1 -> sgn/1
  sgn/1 -> not/1

== system sdbe_10_11/quantize_1/vlbi_2bit/quant14/invcat ==
  b : Inport
  Concat : xbsIndex_r4/Concat  num_inputs=2  dbl_ovrd=off  block_type=concat
  Inverter : xbsIndex_r4/Inverter  en=off  latency=0  dbl_ovrd=off  block_type=inv
  bb : Outport
  wires:
  Concat/1 -> bb/1
  Inverter/1 -> Concat/1
  b/1 -> Concat/2, Inverter/1

== system sdbe_10_11/quantize_1/vlbi_2bit/quant14/is_positive ==
  d : Inport
  Reinterpret : xbsIndex_r4/Reinterpret  force_arith_type=on  arith_type=Unsigned  force_bin_pt=on  bin_pt=0  block_type=reinterpret
  not : xbsIndex_r4/Inverter  en=off  latency=0  dbl_ovrd=off  block_type=inv
  sgn : xbsIndex_r4/Slice  nbits=1  boolean_output=off  mode=Upper Bit Location + Width  bit1=0  base1=MSB of Input  bit0=0  base0=LSB of Input  dbl_ovrd=off  block_type=slice
  q : Outport
  wires:
  sgn/1 -> not/1
  Reinterpret/1 -> sgn/1
  d/1 -> Reinterpret/1
  not/1 -> q/1

== system sdbe_10_11/quantize_1/vlbi_2bit/quant15/invcat ==
  b : Inport
  Concat : xbsIndex_r4/Concat  num_inputs=2  dbl_ovrd=off  block_type=concat
  Inverter : xbsIndex_r4/Inverter  en=off  latency=0  dbl_ovrd=off  block_type=inv
  bb : Outport
  wires:
  b/1 -> Inverter/1, Concat/2
  Inverter/1 -> Concat/1
  Concat/1 -> bb/1

== system sdbe_10_11/quantize_1/vlbi_2bit/quant15/is_positive ==
  d : Inport
  Reinterpret : xbsIndex_r4/Reinterpret  force_arith_type=on  arith_type=Unsigned  force_bin_pt=on  bin_pt=0  block_type=reinterpret
  not : xbsIndex_r4/Inverter  en=off  latency=0  dbl_ovrd=off  block_type=inv
  sgn : xbsIndex_r4/Slice  nbits=1  boolean_output=off  mode=Upper Bit Location + Width  bit1=0  base1=MSB of Input  bit0=0  base0=LSB of Input  dbl_ovrd=off  block_type=slice
  q : Outport
  wires:
  not/1 -> q/1
  d/1 -> Reinterpret/1
  Reinterpret/1 -> sgn/1
  sgn/1 -> not/1

== system sdbe_10_11/quantize_1/vlbi_2bit/quant2/invcat ==
  b : Inport
  Concat : xbsIndex_r4/Concat  num_inputs=2  dbl_ovrd=off  block_type=concat
  Inverter : xbsIndex_r4/Inverter  en=off  latency=0  dbl_ovrd=off  block_type=inv
  bb : Outport
  wires:
  Concat/1 -> bb/1
  Inverter/1 -> Concat/1
  b/1 -> Concat/2, Inverter/1

== system sdbe_10_11/quantize_1/vlbi_2bit/quant2/is_positive ==
  d : Inport
  Reinterpret : xbsIndex_r4/Reinterpret  force_arith_type=on  arith_type=Unsigned  force_bin_pt=on  bin_pt=0  block_type=reinterpret
  not : xbsIndex_r4/Inverter  en=off  latency=0  dbl_ovrd=off  block_type=inv
  sgn : xbsIndex_r4/Slice  nbits=1  boolean_output=off  mode=Upper Bit Location + Width  bit1=0  base1=MSB of Input  bit0=0  base0=LSB of Input  dbl_ovrd=off  block_type=slice
  q : Outport
  wires:
  sgn/1 -> not/1
  Reinterpret/1 -> sgn/1
  d/1 -> Reinterpret/1
  not/1 -> q/1

== system sdbe_10_11/quantize_1/vlbi_2bit/quant3/invcat ==
  b : Inport
  Concat : xbsIndex_r4/Concat  num_inputs=2  dbl_ovrd=off  block_type=concat
  Inverter : xbsIndex_r4/Inverter  en=off  latency=0  dbl_ovrd=off  block_type=inv
  bb : Outport
  wires:
  b/1 -> Inverter/1, Concat/2
  Inverter/1 -> Concat/1
  Concat/1 -> bb/1

== system sdbe_10_11/quantize_1/vlbi_2bit/quant3/is_positive ==
  d : Inport
  Reinterpret : xbsIndex_r4/Reinterpret  force_arith_type=on  arith_type=Unsigned  force_bin_pt=on  bin_pt=0  block_type=reinterpret
  not : xbsIndex_r4/Inverter  en=off  latency=0  dbl_ovrd=off  block_type=inv
  sgn : xbsIndex_r4/Slice  nbits=1  boolean_output=off  mode=Upper Bit Location + Width  bit1=0  base1=MSB of Input  bit0=0  base0=LSB of Input  dbl_ovrd=off  block_type=slice
  q : Outport
  wires:
  not/1 -> q/1
  d/1 -> Reinterpret/1
  Reinterpret/1 -> sgn/1
  sgn/1 -> not/1

== system sdbe_10_11/quantize_1/vlbi_2bit/quant4/invcat ==
  b : Inport
  Concat : xbsIndex_r4/Concat  num_inputs=2  dbl_ovrd=off  block_type=concat
  Inverter : xbsIndex_r4/Inverter  en=off  latency=0  dbl_ovrd=off  block_type=inv
  bb : Outport
  wires:
  Concat/1 -> bb/1
  Inverter/1 -> Concat/1
  b/1 -> Concat/2, Inverter/1

== system sdbe_10_11/quantize_1/vlbi_2bit/quant4/is_positive ==
  d : Inport
  Reinterpret : xbsIndex_r4/Reinterpret  force_arith_type=on  arith_type=Unsigned  force_bin_pt=on  bin_pt=0  block_type=reinterpret
  not : xbsIndex_r4/Inverter  en=off  latency=0  dbl_ovrd=off  block_type=inv
  sgn : xbsIndex_r4/Slice  nbits=1  boolean_output=off  mode=Upper Bit Location + Width  bit1=0  base1=MSB of Input  bit0=0  base0=LSB of Input  dbl_ovrd=off  block_type=slice
  q : Outport
  wires:
  sgn/1 -> not/1
  Reinterpret/1 -> sgn/1
  d/1 -> Reinterpret/1
  not/1 -> q/1

== system sdbe_10_11/quantize_1/vlbi_2bit/quant5/invcat ==
  b : Inport
  Concat : xbsIndex_r4/Concat  num_inputs=2  dbl_ovrd=off  block_type=concat
  Inverter : xbsIndex_r4/Inverter  en=off  latency=0  dbl_ovrd=off  block_type=inv
  bb : Outport
  wires:
  b/1 -> Inverter/1, Concat/2
  Inverter/1 -> Concat/1
  Concat/1 -> bb/1

== system sdbe_10_11/quantize_1/vlbi_2bit/quant5/is_positive ==
  d : Inport
  Reinterpret : xbsIndex_r4/Reinterpret  force_arith_type=on  arith_type=Unsigned  force_bin_pt=on  bin_pt=0  block_type=reinterpret
  not : xbsIndex_r4/Inverter  en=off  latency=0  dbl_ovrd=off  block_type=inv
  sgn : xbsIndex_r4/Slice  nbits=1  boolean_output=off  mode=Upper Bit Location + Width  bit1=0  base1=MSB of Input  bit0=0  base0=LSB of Input  dbl_ovrd=off  block_type=slice
  q : Outport
  wires:
  not/1 -> q/1
  d/1 -> Reinterpret/1
  Reinterpret/1 -> sgn/1
  sgn/1 -> not/1

== system sdbe_10_11/quantize_1/vlbi_2bit/quant6/invcat ==
  b : Inport
  Concat : xbsIndex_r4/Concat  num_inputs=2  dbl_ovrd=off  block_type=concat
  Inverter : xbsIndex_r4/Inverter  en=off  latency=0  dbl_ovrd=off  block_type=inv
  bb : Outport
  wires:
  Concat/1 -> bb/1
  Inverter/1 -> Concat/1
  b/1 -> Concat/2, Inverter/1

== system sdbe_10_11/quantize_1/vlbi_2bit/quant6/is_positive ==
  d : Inport
  Reinterpret : xbsIndex_r4/Reinterpret  force_arith_type=on  arith_type=Unsigned  force_bin_pt=on  bin_pt=0  block_type=reinterpret
  not : xbsIndex_r4/Inverter  en=off  latency=0  dbl_ovrd=off  block_type=inv
  sgn : xbsIndex_r4/Slice  nbits=1  boolean_output=off  mode=Upper Bit Location + Width  bit1=0  base1=MSB of Input  bit0=0  base0=LSB of Input  dbl_ovrd=off  block_type=slice
  q : Outport
  wires:
  sgn/1 -> not/1
  Reinterpret/1 -> sgn/1
  d/1 -> Reinterpret/1
  not/1 -> q/1

== system sdbe_10_11/quantize_1/vlbi_2bit/quant7/invcat ==
  b : Inport
  Concat : xbsIndex_r4/Concat  num_inputs=2  dbl_ovrd=off  block_type=concat
  Inverter : xbsIndex_r4/Inverter  en=off  latency=0  dbl_ovrd=off  block_type=inv
  bb : Outport
  wires:
  b/1 -> Inverter/1, Concat/2
  Inverter/1 -> Concat/1
  Concat/1 -> bb/1

== system sdbe_10_11/quantize_1/vlbi_2bit/quant7/is_positive ==
  d : Inport
  Reinterpret : xbsIndex_r4/Reinterpret  force_arith_type=on  arith_type=Unsigned  force_bin_pt=on  bin_pt=0  block_type=reinterpret
  not : xbsIndex_r4/Inverter  en=off  latency=0  dbl_ovrd=off  block_type=inv
  sgn : xbsIndex_r4/Slice  nbits=1  boolean_output=off  mode=Upper Bit Location + Width  bit1=0  base1=MSB of Input  bit0=0  base0=LSB of Input  dbl_ovrd=off  block_type=slice
  q : Outport
  wires:
  not/1 -> q/1
  d/1 -> Reinterpret/1
  Reinterpret/1 -> sgn/1
  sgn/1 -> not/1

== system sdbe_10_11/quantize_1/vlbi_2bit/quant8/invcat ==
  b : Inport
  Concat : xbsIndex_r4/Concat  num_inputs=2  dbl_ovrd=off  block_type=concat
  Inverter : xbsIndex_r4/Inverter  en=off  latency=0  dbl_ovrd=off  block_type=inv
  bb : Outport
  wires:
  Concat/1 -> bb/1
  Inverter/1 -> Concat/1
  b/1 -> Concat/2, Inverter/1

== system sdbe_10_11/quantize_1/vlbi_2bit/quant8/is_positive ==
  d : Inport
  Reinterpret : xbsIndex_r4/Reinterpret  force_arith_type=on  arith_type=Unsigned  force_bin_pt=on  bin_pt=0  block_type=reinterpret
  not : xbsIndex_r4/Inverter  en=off  latency=0  dbl_ovrd=off  block_type=inv
  sgn : xbsIndex_r4/Slice  nbits=1  boolean_output=off  mode=Upper Bit Location + Width  bit1=0  base1=MSB of Input  bit0=0  base0=LSB of Input  dbl_ovrd=off  block_type=slice
  q : Outport
  wires:
  sgn/1 -> not/1
  Reinterpret/1 -> sgn/1
  d/1 -> Reinterpret/1
  not/1 -> q/1

== system sdbe_10_11/quantize_1/vlbi_2bit/quant9/invcat ==
  b : Inport
  Concat : xbsIndex_r4/Concat  num_inputs=2  dbl_ovrd=off  block_type=concat
  Inverter : xbsIndex_r4/Inverter  en=off  latency=0  dbl_ovrd=off  block_type=inv
  bb : Outport
  wires:
  b/1 -> Inverter/1, Concat/2
  Inverter/1 -> Concat/1
  Concat/1 -> bb/1

== system sdbe_10_11/quantize_1/vlbi_2bit/quant9/is_positive ==
  d : Inport
  Reinterpret : xbsIndex_r4/Reinterpret  force_arith_type=on  arith_type=Unsigned  force_bin_pt=on  bin_pt=0  block_type=reinterpret
  not : xbsIndex_r4/Inverter  en=off  latency=0  dbl_ovrd=off  block_type=inv
  sgn : xbsIndex_r4/Slice  nbits=1  boolean_output=off  mode=Upper Bit Location + Width  bit1=0  base1=MSB of Input  bit0=0  base0=LSB of Input  dbl_ovrd=off  block_type=slice
  q : Outport
  wires:
  not/1 -> q/1
  d/1 -> Reinterpret/1
  Reinterpret/1 -> sgn/1
  sgn/1 -> not/1

== system sdbe_10_11/quantize_2/vlbi_2bit/quant/invcat ==
  b : Inport
  Concat : xbsIndex_r4/Concat  num_inputs=2  dbl_ovrd=off  block_type=concat
  Inverter : xbsIndex_r4/Inverter  en=off  latency=0  dbl_ovrd=off  block_type=inv
  bb : Outport
  wires:
  b/1 -> Inverter/1, Concat/2
  Inverter/1 -> Concat/1
  Concat/1 -> bb/1

== system sdbe_10_11/quantize_2/vlbi_2bit/quant/is_positive ==
  d : Inport
  Reinterpret : xbsIndex_r4/Reinterpret  force_arith_type=on  arith_type=Unsigned  force_bin_pt=on  bin_pt=0  block_type=reinterpret
  not : xbsIndex_r4/Inverter  en=off  latency=0  dbl_ovrd=off  block_type=inv
  sgn : xbsIndex_r4/Slice  nbits=1  boolean_output=off  mode=Upper Bit Location + Width  bit1=0  base1=MSB of Input  bit0=0  base0=LSB of Input  dbl_ovrd=off  block_type=slice
  q : Outport
  wires:
  not/1 -> q/1
  d/1 -> Reinterpret/1
  Reinterpret/1 -> sgn/1
  sgn/1 -> not/1

== system sdbe_10_11/quantize_2/vlbi_2bit/quant1/invcat ==
  b : Inport
  Concat : xbsIndex_r4/Concat  num_inputs=2  dbl_ovrd=off  block_type=concat
  Inverter : xbsIndex_r4/Inverter  en=off  latency=0  dbl_ovrd=off  block_type=inv
  bb : Outport
  wires:
  Concat/1 -> bb/1
  Inverter/1 -> Concat/1
  b/1 -> Concat/2, Inverter/1

== system sdbe_10_11/quantize_2/vlbi_2bit/quant1/is_positive ==
  d : Inport
  Reinterpret : xbsIndex_r4/Reinterpret  force_arith_type=on  arith_type=Unsigned  force_bin_pt=on  bin_pt=0  block_type=reinterpret
  not : xbsIndex_r4/Inverter  en=off  latency=0  dbl_ovrd=off  block_type=inv
  sgn : xbsIndex_r4/Slice  nbits=1  boolean_output=off  mode=Upper Bit Location + Width  bit1=0  base1=MSB of Input  bit0=0  base0=LSB of Input  dbl_ovrd=off  block_type=slice
  q : Outport
  wires:
  sgn/1 -> not/1
  Reinterpret/1 -> sgn/1
  d/1 -> Reinterpret/1
  not/1 -> q/1

== system sdbe_10_11/quantize_2/vlbi_2bit/quant10/invcat ==
  b : Inport
  Concat : xbsIndex_r4/Concat  num_inputs=2  dbl_ovrd=off  block_type=concat
  Inverter : xbsIndex_r4/Inverter  en=off  latency=0  dbl_ovrd=off  block_type=inv
  bb : Outport
  wires:
  b/1 -> Inverter/1, Concat/2
  Inverter/1 -> Concat/1
  Concat/1 -> bb/1

== system sdbe_10_11/quantize_2/vlbi_2bit/quant10/is_positive ==
  d : Inport
  Reinterpret : xbsIndex_r4/Reinterpret  force_arith_type=on  arith_type=Unsigned  force_bin_pt=on  bin_pt=0  block_type=reinterpret
  not : xbsIndex_r4/Inverter  en=off  latency=0  dbl_ovrd=off  block_type=inv
  sgn : xbsIndex_r4/Slice  nbits=1  boolean_output=off  mode=Upper Bit Location + Width  bit1=0  base1=MSB of Input  bit0=0  base0=LSB of Input  dbl_ovrd=off  block_type=slice
  q : Outport
  wires:
  not/1 -> q/1
  d/1 -> Reinterpret/1
  Reinterpret/1 -> sgn/1
  sgn/1 -> not/1

== system sdbe_10_11/quantize_2/vlbi_2bit/quant11/invcat ==
  b : Inport
  Concat : xbsIndex_r4/Concat  num_inputs=2  dbl_ovrd=off  block_type=concat
  Inverter : xbsIndex_r4/Inverter  en=off  latency=0  dbl_ovrd=off  block_type=inv
  bb : Outport
  wires:
  Concat/1 -> bb/1
  Inverter/1 -> Concat/1
  b/1 -> Concat/2, Inverter/1

== system sdbe_10_11/quantize_2/vlbi_2bit/quant11/is_positive ==
  d : Inport
  Reinterpret : xbsIndex_r4/Reinterpret  force_arith_type=on  arith_type=Unsigned  force_bin_pt=on  bin_pt=0  block_type=reinterpret
  not : xbsIndex_r4/Inverter  en=off  latency=0  dbl_ovrd=off  block_type=inv
  sgn : xbsIndex_r4/Slice  nbits=1  boolean_output=off  mode=Upper Bit Location + Width  bit1=0  base1=MSB of Input  bit0=0  base0=LSB of Input  dbl_ovrd=off  block_type=slice
  q : Outport
  wires:
  sgn/1 -> not/1
  Reinterpret/1 -> sgn/1
  d/1 -> Reinterpret/1
  not/1 -> q/1

== system sdbe_10_11/quantize_2/vlbi_2bit/quant12/invcat ==
  b : Inport
  Concat : xbsIndex_r4/Concat  num_inputs=2  dbl_ovrd=off  block_type=concat
  Inverter : xbsIndex_r4/Inverter  en=off  latency=0  dbl_ovrd=off  block_type=inv
  bb : Outport
  wires:
  b/1 -> Inverter/1, Concat/2
  Inverter/1 -> Concat/1
  Concat/1 -> bb/1
